simulink model "feedback_control"  (R2021b)
settings: Solver=VariableStepAuto  StartTime=0.0  StopTime=10.0  RelTol=1e-3
libraries: cstblocks x1
settings Model: Creator=varunsampat  LastModifiedBy=varunsampat

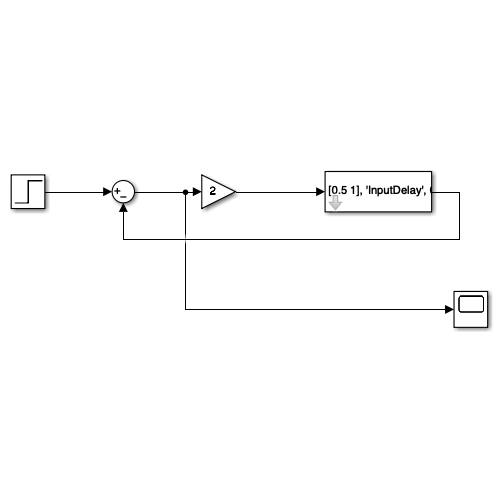
[thumbnail: Simulink's stored preview of the top-level diagram]
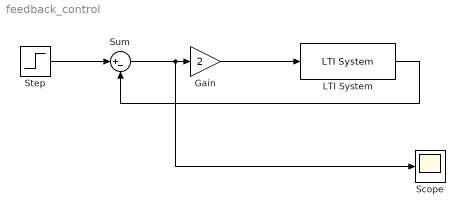
== system feedback_control ==
  Gain : Gain  Gain=2
  LTI System : cstblocks/LTI System  sys=tf(1, [0.5 1], 'InputDelay', 0.5)  IC=[]
  Scope : Scope
  Step : Step  SampleTime=0
  Sum : Sum  Inputs=|+-
  wires:
  Sum/1 -> Scope/1, Gain/1
  Gain/1 -> LTI System/1
  Step/1 -> Sum/1
  LTI System/1 -> Sum/2
